simulink model "ICEV"  (R2021b)
settings: Solver=FixedStepAuto  StartTime=0.0  StopTime=1800  FixedStep=1  RelTol=1e-3
undefined symbols (not defined in the file): gamma, gamma_fd, w_shift
libraries: EnergyConverters x1, DrivingCycle x1, GearSystems x1, GearSystemsControl x1, EnergyStorage x1, VehicleBody x1
settings Model: Creator=dadikozyanaa  LastModifiedBy=dadikozyanaa

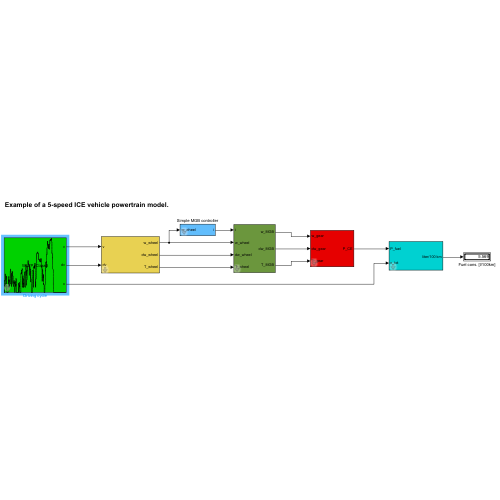
[thumbnail: Simulink's stored preview of the top-level diagram]
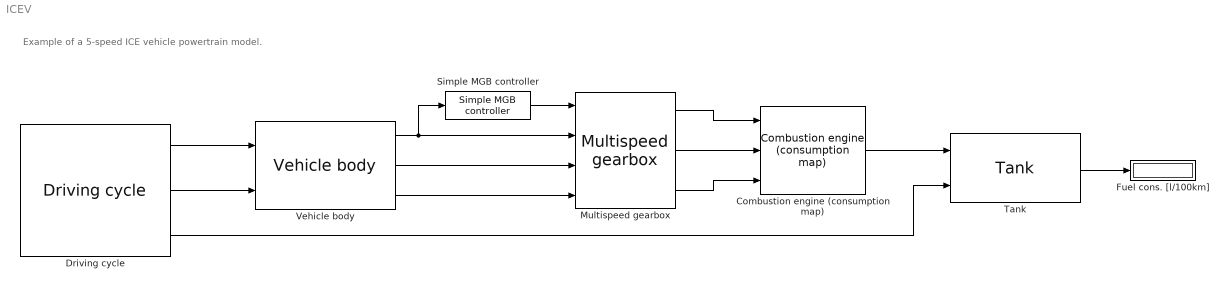
== system ICEV ==
  note: Example of a 5-speed ICE vehicle powertrain model.
  Combustion engine (consumption map) : EnergyConverters/Combustion engine  (consumption map)  Tag=combustion engine  enginetype=Spark ignition  enginenumberCI=119kW  enginenumberSI=102kW  P_aux=Paux_ice  ENABLE_FUEL_CUTOFF=on  T_CE_cutoff=Tcutoff_ice  P_CE_cutoff=Pcutoff_ice  scale_CE=alpha_ice
      settings: SourceProductName=QSS TU/e Toolbox
  Driving cycle : DrivingCycle/Driving cycle  bool_combine=off  cyclenr=Europe: WLTP Class 3  cyclenr2=Europe: EUDC  gradient_speed=0  cyclerep=1  stepsize=1  autostop=on  slope_bool_cycle=off  mode_bool=off  mode_array=0
      settings: SourceProductName=QSS TU/e 4AT030
  Fuel cons. [l/100km] : Display
  Multispeed gearbox : GearSystems/Multispeed gearbox  Tag=transmission  nr_gears=5  i_1=gamma(1)  i_2=gamma(2)  i_3=gamma(3)  i_4=gamma(4)  i_5=gamma(5)  i_6=2.748  i_diff=gamma_fd  e_GT=e_gb  P_GT0=Ploss  w_wheel_min=wem_min
      settings: SourceProductName=QSS TU/e Toolbox
  Simple MGB controller : GearSystemsControl/Simple MGB controller  nr_gears=5  w_shift2=w_shift/gamma(1)/gamma_fd  w_shift3=w_shift/gamma(2)/gamma_fd  w_shift4=w_shift/gamma(3)/gamma_fd  w_shift5=w_shift/gamma(4)/gamma_fd  w_shift6=1e10
      settings: SourceProductName=QSS TU/e 4AT030
  Tank : EnergyStorage/Tank  Tag=tank  fuel=Gasoline  flag_cold_start=on
      settings: SourceProductName=QSS TU/e 4AT030
  Vehicle body : VehicleBody/Vehicle body  m_f=mv  mt2m_f=J_rot  A_f=Af  d_wheel=dw  cw=cd  mu=cr  f_r=f_r  slope_bool=off
      settings: SourceProductName=QSS TU/e 4AT030
  wires:
  Driving cycle/1 -> Vehicle body/1
  Driving cycle/2 -> Vehicle body/2
  Tank/1 -> Fuel cons. [l/100km]/1
  Multispeed gearbox/1 -> Combustion engine (consumption map)/1
  Multispeed gearbox/2 -> Combustion engine (consumption map)/2
  Multispeed gearbox/3 -> Combustion engine (consumption map)/3
  Combustion engine (consumption map)/1 -> Tank/1
  Vehicle body/1 -> Multispeed gearbox/2, Simple MGB controller/1
  Simple MGB controller/1 -> Multispeed gearbox/1
  Vehicle body/2 -> Multispeed gearbox/3
  Vehicle body/3 -> Multispeed gearbox/4
  Driving cycle/3 -> Tank/2
